simulink model "switch_controller"  (R2020a)
settings: Solver=VariableStepAuto  StartTime=0.0  StopTime=0.05  RelTol=1e-3
undefined symbols (not defined in the file): G, K, us, xs
libraries: powerlib x11, eeLuenbergerObserver x2, powerlib_meascontrol x1, eeGeneralControl x1
settings Model: Creator=Slash  LastModifiedBy=Slash

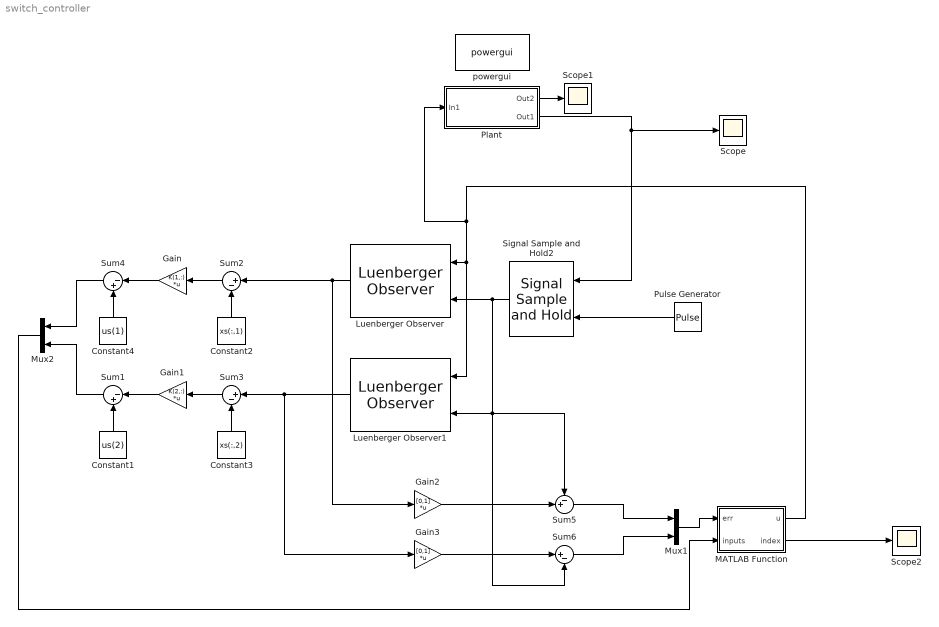
== system switch_controller ==
  Constant1 : Constant  Value=us(2)
  Constant2 : Constant  Value=xs(:,1)
  Constant3 : Constant  Value=xs(:,2)
  Constant4 : Constant  Value=us(1)
  Gain : Gain  Gain=K(1,:)  Multiplication=Matrix(K*u)
  Gain1 : Gain  Gain=K(2,:)  Multiplication=Matrix(K*u)
  Gain2 : Gain  Gain=[0,1]  Multiplication=Matrix(K*u)
  Gain3 : Gain  Gain=[0,1]  Multiplication=Matrix(K*u)
  Luenberger Observer : eeLuenbergerObserver/Luenberger Observer  StateSpaceType=Discrete-time  Ad=G(:,:,1,1).A  Bd=G(:,:,1,1).B  Cd=[0,1]  Dd=0  A=1  B=1  C=1  D=1  ObserverDesign=Desired eigenvalues  Ld=[0;0]  DesiredEigenvalues=[0.2,0.21]  x0=[0,0]  Tsd=0.1  Ts=0.001
      settings: SourceProductBaseCode=PS
  Luenberger Observer1 : eeLuenbergerObserver/Luenberger Observer  StateSpaceType=Discrete-time  Ad=G(:,:,2,1).A  Bd=G(:,:,2,1).B  Cd=[0,1]  Dd=0  A=1  B=1  C=1  D=1  ObserverDesign=Desired eigenvalues  Ld=[0;0]  DesiredEigenvalues=[0.2,0.21]  x0=[0,0]  Tsd=0.1  Ts=0.001
      settings: SourceProductBaseCode=PS
  MATLAB Function : MATLAB Function  TreatAsAtomicUnit=on
  Mux1 : Mux  Inputs=2
  Mux2 : Mux  Inputs=2
  Plant : Subsystem
  Pulse Generator : DiscretePulseGenerator  PulseType=Time based  Period=0.001
  Scope : Scope
  Scope1 : Scope
  Scope2 : Scope
  Signal Sample and Hold2 : eeGeneralControl/Signal Sample and Hold  LabelModeActiveChoice=Discrete  x0=0  Ts=0.001
      settings: SourceProductBaseCode=PS
  Sum1 : Sum  Inputs=|-+
  Sum2 : Sum  Inputs=|+-
  Sum3 : Sum  Inputs=|+-
  Sum4 : Sum  Inputs=|-+
  Sum5 : Sum  Inputs=-+|
  Sum6 : Sum  Inputs=|+-
  powergui : powerlib/powergui  Priority=1  SimulationMode=Continuous  SampleTime=50e-6  frequency=60  Iterations=50  frequencyindice=0  Pbase=100e6  ErrMax=1e-4  UnitsV=kV  UnitsW=MW  buscounter=0  FunctionMessages=off  echomessages=off  EnableUseOfTLC=off  CurrentSourceSwitches=off  DisableSnubberDevices=off  DisableRonSwitches=off  DisableVfSwitches=off  DisplayEquations=off  AutomaticDiscreteSolvers=off  SolverType=Tustin/Backward Euler (TBE)  Interpol=off  ExternalGateDelay=off  methode=off  Ts=100  x0status=blocks  SPID=on  SwTol=0  HookPort=off  NonlinearTolerance=1e-4  nMaxIteration=100  ContinueOnMaxIteration=off  RestoreLinks=warning  ResistiveCurrentMeasurement=off  Frange=[0:2:500]  Ylog=off  Xlog=on  ShowGrid=off  save=off  variable=ZData  structure=0  ZoomFFT=off  StartTime=0.0  cycles=1  DisplayStyle=1  fundamental=60  FreqAxis=off  MaxFrequency=1000  frequencyindicesteady=1  RmsSteady=1  display=off
  wires:
  Signal Sample and Hold2/1 -> Sum6/2, Luenberger Observer1/2, Sum5/1, Luenberger Observer/2
  Pulse Generator/1 -> Signal Sample and Hold2/2
  Plant/2(Out1) -> Signal Sample and Hold2/1, Scope/1
  Plant/1(Out2) -> Scope1/1
  Luenberger Observer/1 -> Gain2/1, Sum2/1
  Sum2/1 -> Gain/1
  Constant2/1 -> Sum2/2
  Luenberger Observer1/1 -> Gain3/1, Sum3/1
  Constant3/1 -> Sum3/2
  Sum3/1 -> Gain1/1
  Gain/1 -> Sum4/1
  Constant4/1 -> Sum4/2
  Gain1/1 -> Sum1/1
  MATLAB Function/1(u) -> Plant/1(In1), Luenberger Observer/1, Luenberger Observer1/1
  Gain3/1 -> Sum6/1
  Gain2/1 -> Sum5/2
  Sum5/1 -> Mux1/1
  Sum6/1 -> Mux1/2
  Mux1/1 -> MATLAB Function/1(err)
  Sum4/1 -> Mux2/1
  Sum1/1 -> Mux2/2
  Mux2/1 -> MATLAB Function/2(inputs)
  MATLAB Function/2(index) -> Scope2/1
  Constant1/1 -> Sum1/2

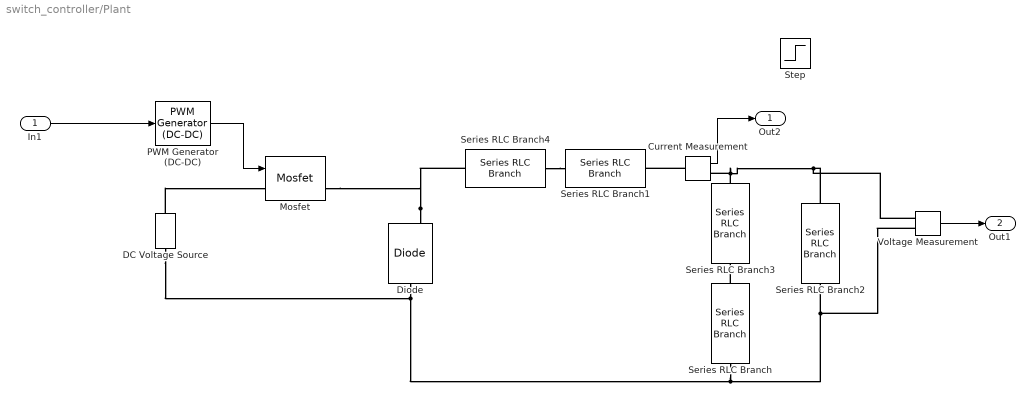
== system switch_controller/Plant ==
  In1 : Inport
  Current Measurement : powerlib/Measurements/Current Measurement  PhasorSimulation=off  OutputType=Complex  PSBequivalent=0
  DC Voltage Source : powerlib/Electrical Sources/DC Voltage Source  Amplitude=15  Measurements=None
  Diode : powerlib/Power Electronics/Diode  Ron=0.001  Lon=0  Vf=0.1  IC=0  UseSnubber=0  Rs=500  Cs=250e-9  Measurements=on
  Mosfet : powerlib/Power Electronics/Mosfet  Ron=0.05  Lon=0  Rd=0.01  Vfd=0  IC=0  Rs=1e5  Cs=inf  Measurements=on
  PWM Generator (DC-DC) : powerlib_meascontrol/Pulse & Signal Generators/PWM Generator (DC-DC)  Fsw=20000  Ts=0
  Series RLC Branch : powerlib/Elements/Series RLC Branch  LConnTagsString=__new0  RConnTagsString=__new0  BranchType=C  Resistance=1  Inductance=1e-3  SetiL0=off  InitialCurrent=0  Capacitance=56e-6  Setx0=off  InitialVoltage=0  Measurements=None
  Series RLC Branch1 : powerlib/Elements/Series RLC Branch  LConnTagsString=__new0  RConnTagsString=__new0  BranchType=L  Resistance=1  Inductance=10e-3  SetiL0=off  InitialCurrent=0  Capacitance=1e-6  Setx0=off  InitialVoltage=0  Measurements=None
  Series RLC Branch2 : powerlib/Elements/Series RLC Branch  LConnTagsString=__new0  RConnTagsString=__new0  BranchType=R  Resistance=100  Inductance=1e-3  SetiL0=off  InitialCurrent=0  Capacitance=1e-6  Setx0=off  InitialVoltage=0  Measurements=None
  Series RLC Branch3 : powerlib/Elements/Series RLC Branch  LConnTagsString=__new0  RConnTagsString=__new0  BranchType=R  Resistance=0.33  Inductance=1e-3  SetiL0=off  InitialCurrent=0  Capacitance=1e-6  Setx0=off  InitialVoltage=0  Measurements=None
  Series RLC Branch4 : powerlib/Elements/Series RLC Branch  LConnTagsString=__new0  RConnTagsString=__new0  BranchType=R  Resistance=1.6  Inductance=1e-3  SetiL0=off  InitialCurrent=0  Capacitance=1e-6  Setx0=off  InitialVoltage=0  Measurements=None
  Step : Step  Time=0.05  Before=100  After=18  SampleTime=0
  Voltage Measurement : powerlib/Measurements/Voltage Measurement  PhasorSimulation=off  OutputType=Complex  PSBequivalent=0
  Out2 : Outport
  Out1 : Outport  Port=2
  wires:
  Voltage Measurement/1 -> Out1/1
  PWM Generator (DC-DC)/1 -> Mosfet/1
  In1/1 -> PWM Generator (DC-DC)/1
  Current Measurement/1 -> Out2/1
  connections:
  Diode/LConn1 -- DC Voltage Source/LConn1 -- Series RLC Branch/RConn1 -- Voltage Measurement/LConn2 -- Series RLC Branch2/RConn1
  Diode/RConn1 -- Series RLC Branch4/RConn1 -- Mosfet/RConn1
  Series RLC Branch3/LConn1 -- Current Measurement/RConn1 -- Series RLC Branch2/LConn1 -- Voltage Measurement/LConn1
  Series RLC Branch/LConn1 -- Series RLC Branch3/RConn1
  DC Voltage Source/RConn1 -- Mosfet/LConn1
  Series RLC Branch4/LConn1 -- Series RLC Branch1/LConn1
  Current Measurement/LConn1 -- Series RLC Branch1/RConn1

== matlab function switch_controller/MATLAB Function ==
  data: err input size=2; u output size=1; inputs input size=2; index output
function [u,index] = fcn(err, inputs)
    err = err.^2;
    [~,index]=min(err);
    u = inputs(index);
end
